simulink model "n2o_pressure"  (R2026a)
settings: Solver=VariableStepAuto
libraries: simulink x2
settings Model: Creator=aslan  LastModifiedBy=aslan

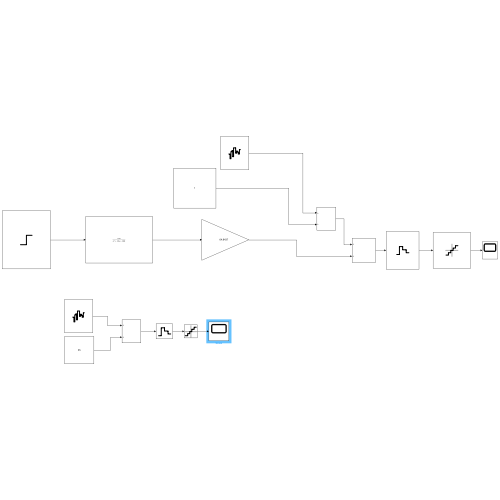
[thumbnail: Simulink's stored preview of the top-level diagram]
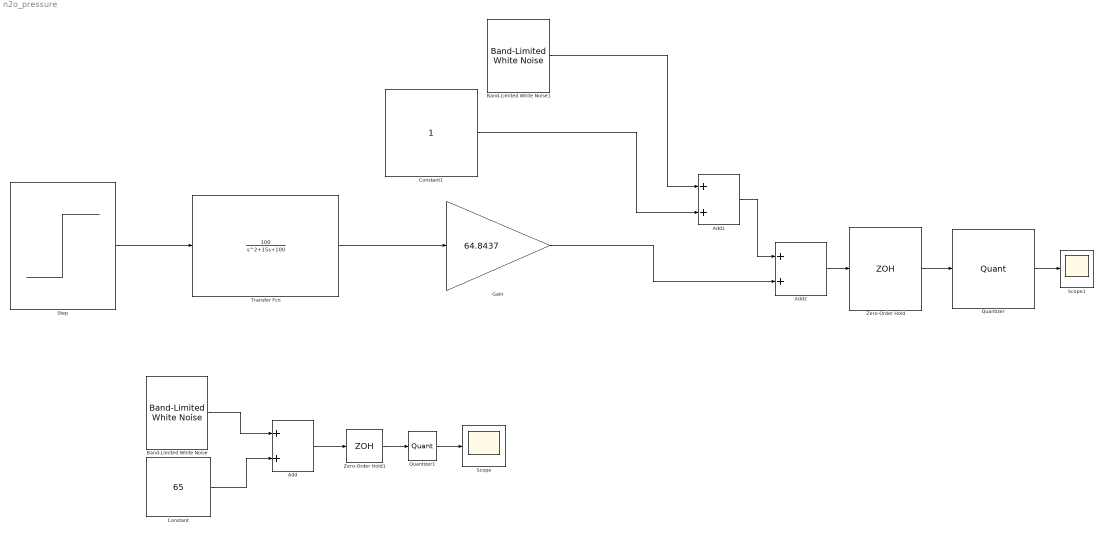
== system n2o_pressure ==
  Add : Sum
  Add1 : Sum
  Add2 : Sum
  Band-Limited White Noise : simulink/Sources/Band-Limited White Noise  Cov=[0.0001]  Ts=0.1  seed=[23341]
  Band-Limited White Noise1 : simulink/Sources/Band-Limited White Noise  Cov=[0.0001]  Ts=0.1  seed=[23341]
  Constant : Constant  Value=65
  Constant1 : Constant
  Gain : Gain  Gain=64.8437
  Quantizer : Quantizer  QuantizationInterval=0.0015
  Quantizer1 : Quantizer
  Scope : Scope
      settings: ActiveDisplayYMinimum=55.744080004145282  ActiveDisplayYMaximum=73.8846695733063
  Scope1 : Scope
      settings: ActiveDisplayYMinimum=-24.148481627969698  ActiveDisplayYMaximum=107.91720441543661
  Step : Step  Time=1.0  SampleTime=0
  Transfer Fcn : TransferFcn  Numerator=[100]  Denominator=[1 15 100]
  Zero-Order Hold : ZeroOrderHold  SampleTime=0.001
  Zero-Order Hold1 : ZeroOrderHold  SampleTime=-1
  wires:
  Constant/1 -> Add/2
  Band-Limited White Noise/1 -> Add/1
  Step/1 -> Transfer Fcn/1
  Transfer Fcn/1 -> Gain/1
  Add2/1 -> Zero-Order Hold/1
  Zero-Order Hold/1 -> Quantizer/1
  Add/1 -> Zero-Order Hold1/1
  Zero-Order Hold1/1 -> Quantizer1/1
  Quantizer1/1 -> Scope/1
  Constant1/1 -> Add1/2
  Band-Limited White Noise1/1 -> Add1/1
  Add1/1 -> Add2/1
  Gain/1 -> Add2/2
  Quantizer/1 -> Scope1/1
